simulink model "Tricopter_Controlled"  (R2012b)
settings: Solver=ode3  StartTime=0.0  StopTime=inf  FixedStep=T_sim  MaxStep=0.01  RelTol=1e-5
values from neighbouring files (symbols this model uses):
  A_l_max_x = sqrt( (Max_Thrust*3/m)^2  -  g^2  )    [Run3Copter.m]
  A_x = 0.015    [SetupComplete.m]
  A_y = A_x    (= 0.015)    [SetupComplete.m]
  A_z = 0.16    [SetupComplete.m]
  A_z_max = Max_Thrust*3/m    [Run3Copter.m]
  Alt_0 = input(' Give the initial altitude (m): ')    [Run3Copter.m]
  C_x = 1.2    [SetupComplete.m]
  C_y = C_x    (= 1.2)    [SetupComplete.m]
  C_z = 2.2    [SetupComplete.m]
  CG_0 = [0,0,0.02]'    [SetupComplete.m]
  epsilon = 0.01    [Run3Copter.m]
  eta_1 = deg2rad(-2)    [Run3Copter.m]
  eta_23 = 0    [Run3Copter.m]
  g = 9.81    [SetupComplete.m]
  h_M = 0.064    [SetupComplete.m]
  I_BAC_0 = [ Ix,0,Ixz;0,Iy,0;Ixz,0,Iz]    [SetupComplete.m]
  Initial_Omegas = Omega_hover    [Run3Copter.m]
  Initial_Torques = Torque_hover    [Run3Copter.m]
  Ix = 0.0552    [SetupComplete.m]
  Iy = 0.0552    [SetupComplete.m]
  Iz = 0.11    [SetupComplete.m]
  l = 0.345    [SetupComplete.m]
  l_arm = 0.264    [SetupComplete.m]
  latitude = 52.0733    [Run3Copter.m]
  longitude = 0.6278    [Run3Copter.m]
  m = 3.51    [SetupComplete.m]
  m_0 = 2.61    [SetupComplete.m]
  m_M = 0.300    (= 0.3)    [SetupComplete.m]
  rho = 1.15    [SetupComplete.m]
  Rotation_sign = [ 1,-1,-1]    [SetupComplete.m]
  T_sim = 0.01    [Run3Copter.m]
  throtle_1 = throtle_23/cos(eta_1)    [Run3Copter.m]
  throtle_23 = 0.745    [Run3Copter.m]
  v_i0 = sqrt( 1/3*m*g/(2*rho*pi*R^2)  )    [SetupComplete.m]
undefined symbols (not defined in the file or in its folder): DOWN_0, Earth, EAST_0, Newton, NORTH_0, P_0, Q_0, R_0, Raphson, U_0, V_0, W_0, WGS84
libraries: Adaptive_FaultTolerantControl x24, simulink_extras x11, XXCopter_C x7, XXCopter x5, aerolibfltsims x3, XXCopter_Control x2, qcatlib x1, aerolibconvert2 x1, aerolibtransform2 x1, aerolibanimutils x1, aerolibobsolete x1, simulink x1
(part 2 of 3)

== system Tricopter_Controlled/Inner Controller/P Controller ==
  note: These limits are wrong?
  note: Limits here for the maximum asymetrical thortle deflection
  Accels ref (m/s^2) : Inport
  Phi_ref (rad) : Inport  Port=2
  Theta_ref (rad) : Inport  Port=3
  Yaw_ref (rad) : Inport  Port=4
  All meas : Inport  Port=5
  Attitude Controller : Subsystem
  Body Rates Controller : Subsystem
  Bus Selector : BusSelector  OutputSignals=Meas.Euler meas (rad)
  Demux : Demux  Outputs=3
  MATLAB Function : MATLAB Function  TreatAsAtomicUnit=on
      settings: PermitHierarchicalResolution=ParametersOnly
  Mux : Mux  Inputs=2
  Saturation : Saturate  UpperLimit=[0.4,0.4,0.1]'  LowerLimit=-[0.4,0.4,0.1]'
  Saturation1 : Saturate  UpperLimit=deg2rad(45)/5*[2,2,1]'  LowerLimit=-deg2rad(45)/5*[2,2,1]'
  Accs_Ang_acc des : Outport
  wires:
  Accels ref (m/s^2)/1 -> Mux/1
  Body Rates Controller/1(Angular acc des (rad/s^2)) -> Saturation/1
  MATLAB Function/1(Omega) -> Demux/1
  Mux/1 -> Accs_Ang_acc des/1
  Attitude Controller/1(Euler_dot des (rad/s)) -> Saturation1/1
  All meas/1 -> Attitude Controller/4(All_meas), Body Rates Controller/4(All_meas), Bus Selector/1
  Phi_ref (rad)/1 -> Attitude Controller/1(phi_ref)
  Yaw_ref (rad)/1 -> Attitude Controller/3(psi_ref)
  Theta_ref (rad)/1 -> Attitude Controller/2(theta_ref)
  Bus Selector/1 -> MATLAB Function/2(euler_ang)  "<Euler meas (rad)>"
  Demux/1 -> Body Rates Controller/1(p_ref)
  Demux/2 -> Body Rates Controller/2(q_ref)
  Demux/3 -> Body Rates Controller/3(r_ref)
  Saturation/1 -> Mux/2
  Saturation1/1 -> MATLAB Function/1(ang_dot)

== system Tricopter_Controlled/Inner Controller/PI Controller ==
  note: Limits here for the maximum asymetrical thortle deflection
  Accels ref (m/s^2) : Inport
  Phi_ref (rad) : Inport  Port=2
  Theta_ref (rad) : Inport  Port=3
  Yaw_ref (rad) : Inport  Port=4
  All meas : Inport  Port=5
  Attitude Controller : Subsystem
  Body Rates Controller : Subsystem
  Bus Selector : BusSelector  OutputSignals=Meas.Euler meas (rad)
  Demux : Demux  Outputs=3
  Limits in Ang accel : Subsystem  TreatAsAtomicUnit=on
  MATLAB Function : MATLAB Function  TreatAsAtomicUnit=on
      settings: PermitHierarchicalResolution=ParametersOnly
  Mux : Mux  Inputs=2
  Saturation1 : Saturate  UpperLimit=deg2rad(45)*[1,1,0.5]'  LowerLimit=-deg2rad(45)*[1,1,0.5]'
  keep -pi/pi1 : Subsystem
  keep -pi/pi2 : Subsystem
  keep -pi/pi3 : Subsystem
  Accs_Ang_acc des : Outport
  wires:
  Limits in Ang accel/1(ang Ace des) -> Mux/2
  Demux/3 -> Body Rates Controller/3(r_ref)
  Demux/2 -> Body Rates Controller/2(q_ref)
  Demux/1 -> Body Rates Controller/1(p_ref)
  Bus Selector/1 -> Limits in Ang accel/2(Euler meas), MATLAB Function/2(euler_ang)  "<Euler meas (rad)>"
  Theta_ref (rad)/1 -> keep -pi/pi2/1(in (rad))
  Yaw_ref (rad)/1 -> keep -pi/pi3/1(in (rad))
  Phi_ref (rad)/1 -> keep -pi/pi1/1(in (rad))
  All meas/1 -> Body Rates Controller/4(All_meas), Bus Selector/1, Attitude Controller/4(All_meas)
  Mux/1 -> Accs_Ang_acc des/1
  MATLAB Function/1(Omega) -> Demux/1
  Accels ref (m/s^2)/1 -> Mux/1
  Body Rates Controller/1(Angular acc des (rad/s^2)) -> Limits in Ang accel/1(Ang Ace des)
  keep -pi/pi1/1(out (rad)) -> Attitude Controller/1(phi_ref)
  keep -pi/pi2/1(out (rad)) -> Attitude Controller/2(theta_ref)
  keep -pi/pi3/1(out (rad)) -> Attitude Controller/3(psi_ref)
  Attitude Controller/1(Euler_dot des (rad/s)) -> Saturation1/1
  Saturation1/1 -> MATLAB Function/1(ang_dot)

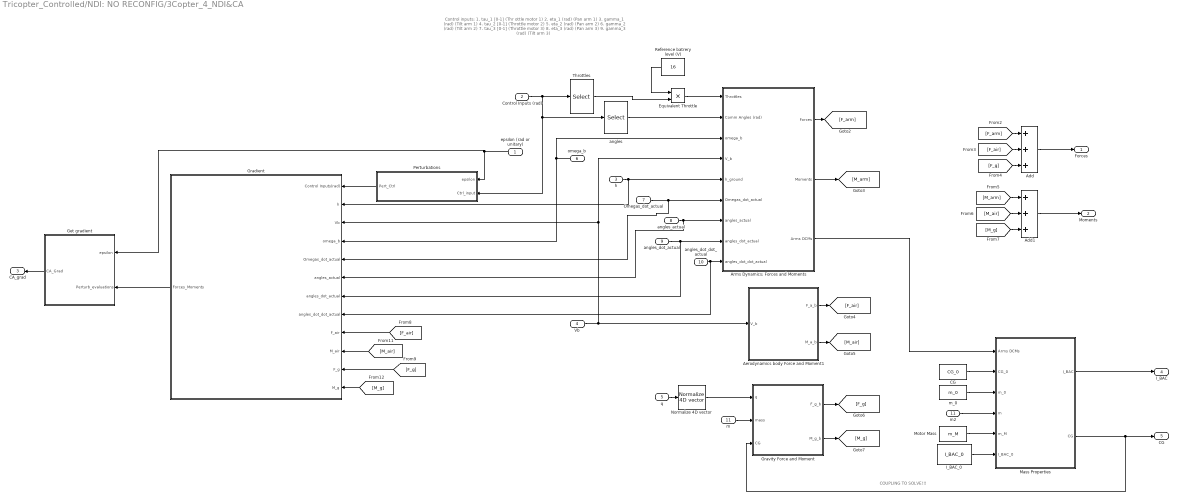
== system Tricopter_Controlled/NDI: NO RECONFIG/3Copter_4_NDI&CA ==
  note: Control inputs:
      | 1. tau_1 [0-1] (Thr ottle motor 1)
      | 2. eta_1 (rad)  (Pan arm 1)
      | 3. gamma_1 (rad)  (Tilt arm 1)
      |
      | 4. tau_2 [0-1] (Throttle motor 2)
      | 5. eta_2 (rad)  (Pan arm 2)
      | 6. gamma_2 (rad)  (Tilt arm 2)
      |
      | 7. tau_3 [0-1] (Throttle motor 3)
      | 8. eta_3 (rad)  (Pan arm  3)
      | 9. gamma_3 (rad)  (Tilt arm 3)
  note: COUPLING TO SOLVE!!!
  "epsilon (rad or unitary) " : Inport
  Control Inputs (rad) : Inport  Port=2
  h : Inport  Port=3
  Vb : Inport  Port=4
  q : Inport  Port=5
  omega_b : Inport  Port=6
  Omegas_dot_actual : Inport  Port=7
  angles_actual : Inport  Port=8
  angles_dot_actual : Inport  Port=9
  angles_dot_dot_actual : Inport  Port=10
  " m" : Inport  Port=11
  Add : Sum  Inputs=+++
  Add1 : Sum  Inputs=+++
  Aerodynamics body Force and Moment1 : MATLAB Function  TreatAsAtomicUnit=on
      settings: PermitHierarchicalResolution=ParametersOnly
  Arms Dynamics: Forces and Moments : Subsystem  TreatAsAtomicUnit=on
  CG : Constant  Value=CG_0
  Equivalent Throttle : Product  Inputs=**
  Get gradient : MATLAB Function  TreatAsAtomicUnit=on
      settings: PermitHierarchicalResolution=ParametersOnly
  Gradient : Subsystem  TreatAsAtomicUnit=on
  Gravity Force and Moment : MATLAB Function  TreatAsAtomicUnit=on
      settings: PermitHierarchicalResolution=ParametersOnly
  I_BAC_0 : Constant  Value=I_BAC_0
  Mass Properties : Subsystem  TreatAsAtomicUnit=on
  Motor Mass : Constant  Value=m_M
  Normalize 4D vector : XXCopter/Normalize 4D vector
  Perturbations : MATLAB Function  TreatAsAtomicUnit=on
      settings: PermitHierarchicalResolution=ParametersOnly
  Reference batrery level (V) : Constant  Value=16
  Throttles : Selector  IndexMode=Zero-based  InputPortWidth=9  Indices=[0,3,6]
  "angles " : Selector  IndexMode=Zero-based  InputPortWidth=9  Indices=[1,2,4,5,7,8]
  m2 : InportShadow  Port=11
  m_0 : Constant  Value=m_0
  Forces : Outport
  Moments : Outport  Port=2
  CA_grad : Outport  Port=3
  I_BAC : Outport  Port=4
  "CG " : Outport  Port=5
  wires:
  Get gradient/1(CA_Grad) -> CA_grad/1
  "epsilon (rad or unitary) "/1 -> Perturbations/1(epsilon), Get gradient/1(epsilon)
  Perturbations/1(Pert_Ctrl) -> Gradient/1("Control Inputs(rad) ")
  Gradient/1(Forces_Moments) -> Get gradient/2(Perturb_evaluations)
  Mass Properties/1(I_BAC) -> I_BAC/1
  [F_g] -> Gradient/11(F_g)
  [F_air] -> Gradient/9(F_air)
  [M_air] -> Gradient/10(M_air)
  [M_g] -> Gradient/12(M_g)
  Normalize 4D vector/1 -> Gravity Force and Moment/1(q)
  angles_dot_actual/1 -> Arms Dynamics: Forces and Moments/8(angles_dot_actual), Gradient/7(angles_dot_actual)
  Omegas_dot_actual/1 -> Gradient/5(Omegas_dot_actual), Arms Dynamics: Forces and Moments/6(Omegas_dot_actual)
  q/1 -> Normalize 4D vector/1
  Add1/1 -> Moments/1
  Reference batrery level (V)/1 -> Equivalent Throttle/1
  Equivalent Throttle/1 -> Arms Dynamics: Forces and Moments/1(Throttles)
  Mass Properties/2(CG) -> Gravity Force and Moment/3(CG), "CG "/1
  Add/1 -> Forces/1
  m2/1 -> Mass Properties/4(m)
  m_0/1 -> Mass Properties/3(m_0)
  I_BAC_0/1 -> Mass Properties/6(I_BAC_0)
  Motor Mass/1 -> Mass Properties/5(m_M)
  CG/1 -> Mass Properties/2(CG_0)
  Arms Dynamics: Forces and Moments/3(Arms DCMs) -> Mass Properties/1(Arms DCMs)
  Control Inputs (rad)/1 -> Throttles/1, Perturbations/2(Ctrl_input), "angles "/1
  Throttles/1 -> Equivalent Throttle/2
  [M_air] -> Add1/2
  [M_g] -> Add1/3
  [M_arm] -> Add1/1
  [F_g] -> Add/3
  [F_air] -> Add/2
  [F_arm] -> Add/1
  Gravity Force and Moment/2(M_g_b) -> [M_g]
  Gravity Force and Moment/1(F_g_b) -> [F_g]
  Aerodynamics body Force and Moment1/2(M_a_b) -> [M_air]
  Aerodynamics body Force and Moment1/1(F_a_b) -> [F_air]
  Arms Dynamics: Forces and Moments/2(Moments) -> [M_arm]
  Arms Dynamics: Forces and Moments/1(Forces) -> [F_arm]
  h/1 -> Gradient/2(h), Arms Dynamics: Forces and Moments/5(h_ground)
  " m"/1 -> Gravity Force and Moment/2(mass)
  omega_b/1 -> Gradient/4(omega_b), Arms Dynamics: Forces and Moments/3(omega_b)
  Vb/1 -> Aerodynamics body Force and Moment1/1(V_b), Arms Dynamics: Forces and Moments/4(V_b), Gradient/3(Vb)
  angles_actual/1 -> Gradient/6(angles_actual), Arms Dynamics: Forces and Moments/7(angles_actual)
  "angles "/1 -> Arms Dynamics: Forces and Moments/2(Comm Angles (rad))
  angles_dot_dot_actual/1 -> Gradient/8(angles_dot_dot_actual), Arms Dynamics: Forces and Moments/9(angles_dot_dot_actual)

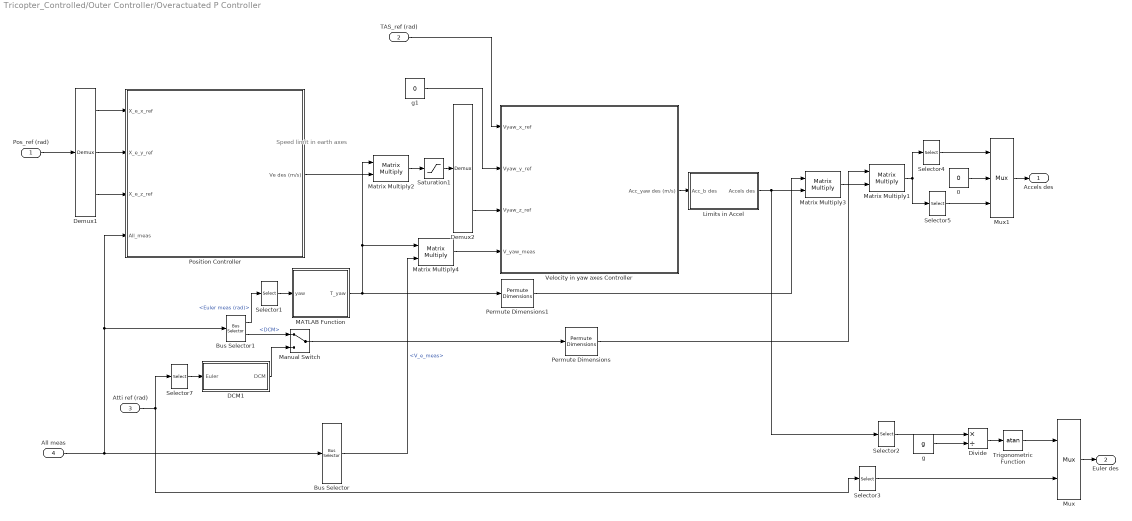
== system Tricopter_Controlled/Outer Controller/Overactuated P Controller ==
  note: Speed limit
      | in earth axes
  Pos_ref (rad) : Inport
  TAS_ref (rad) : Inport  Port=2
  Atti ref (rad) : Inport  Port=3
  All meas : Inport  Port=4
  0 : Constant  Value=0
  Bus Selector : BusSelector  OutputSignals=Meas.V_e_meas
  Bus Selector1 : BusSelector  OutputSignals=Meas.Euler meas (rad),DCM
  DCM1 : Subsystem  TreatAsAtomicUnit=on
  Demux1 : Demux  Outputs=3
  Demux2 : Demux  Outputs=3
  Divide : Product  Inputs=*/
  Limits in Accel : Subsystem  TreatAsAtomicUnit=on
  MATLAB Function : MATLAB Function  TreatAsAtomicUnit=on
      settings: PermitHierarchicalResolution=ParametersOnly
  Manual Switch : ManualSwitch
  Matrix Multiply{1..4} (4 alike) : Product  Multiplication=Matrix(*)
  Mux : Mux  Inputs=2
  Mux1 : Mux  Inputs=3
  Permute Dimensions : PermuteDimensions
  Permute Dimensions1 : PermuteDimensions
  Position Controller : Subsystem
  Saturation1 : Saturate  UpperLimit=[10,10,v_i0]  LowerLimit=-[10,10,v_i0*2]
  Selector1 : Selector  InputPortWidth=3  Indices=3
  Selector2 : Selector  InputPortWidth=3  Indices=2
  Selector3 : Selector  InputPortWidth=3  Indices=[2,3]
  Selector4 : Selector  InputPortWidth=3
  Selector5 : Selector  InputPortWidth=3  Indices=3
  Selector7 : Selector  InputPortWidth=3  Indices=[3 2 1]
  Trigonometric Function : Trigonometry  Operator=atan
  Velocity in yaw axes Controller : Subsystem
  g : Constant  Value=g
  g1 : Constant  Value=0
  Accels des : Outport
  Euler des : Outport  Port=2
  wires:
  Demux2/3 -> Velocity in yaw axes Controller/3(Vyaw_z_ref)
  Atti ref (rad)/1 -> Selector3/1, Selector7/1
  All meas/1 -> Position Controller/4(All_meas), Bus Selector1/1, Bus Selector/1
  Pos_ref (rad)/1 -> Demux1/1
  Demux1/3 -> Position Controller/3(X_e_z_ref)
  Demux1/2 -> Position Controller/2(X_e_y_ref)
  Demux1/1 -> Position Controller/1(X_e_x_ref)
  Selector7/1 -> DCM1/1(Euler)
  DCM1/1(DCM) -> Manual Switch/2
  Bus Selector1/2 -> Manual Switch/1  "<DCM>"
  Velocity in yaw axes Controller/1(Acc_yaw des (m/s)) -> Limits in Accel/1(Acc_b des)
  Matrix Multiply1/1 -> Selector4/1, Selector5/1
  Manual Switch/1 -> Permute Dimensions/1
  Permute Dimensions/1 -> Matrix Multiply1/1
  Selector1/1 -> MATLAB Function/1(yaw)
  Bus Selector1/1 -> Selector1/1  "<Euler meas (rad)>"
  Position Controller/1(Ve des (m/s)) -> Matrix Multiply2/2
  Saturation1/1 -> Demux2/1
  Limits in Accel/1(Accels des) -> Selector2/1, Matrix Multiply3/2
  MATLAB Function/1(T_yaw) -> Permute Dimensions1/1, Matrix Multiply2/1, Matrix Multiply4/1
  Matrix Multiply2/1 -> Saturation1/1
  Matrix Multiply3/1 -> Matrix Multiply1/2
  Permute Dimensions1/1 -> Matrix Multiply3/1
  Matrix Multiply4/1 -> Velocity in yaw axes Controller/4(V_yaw_meas)
  Bus Selector/1 -> Matrix Multiply4/2  "<V_e_meas>"
  TAS_ref (rad)/1 -> Velocity in yaw axes Controller/1(Vyaw_x_ref)
  Selector2/1 -> Divide/1
  g/1 -> Divide/2
  Divide/1 -> Trigonometric Function/1
  Mux/1 -> Euler des/1
  Selector3/1 -> Mux/2
  Mux1/1 -> Accels des/1
  Selector4/1 -> Mux1/1
  Selector5/1 -> Mux1/3
  0/1 -> Mux1/2
  Trigonometric Function/1 -> Mux/1
  g1/1 -> Velocity in yaw axes Controller/2(Vyaw_y_ref)

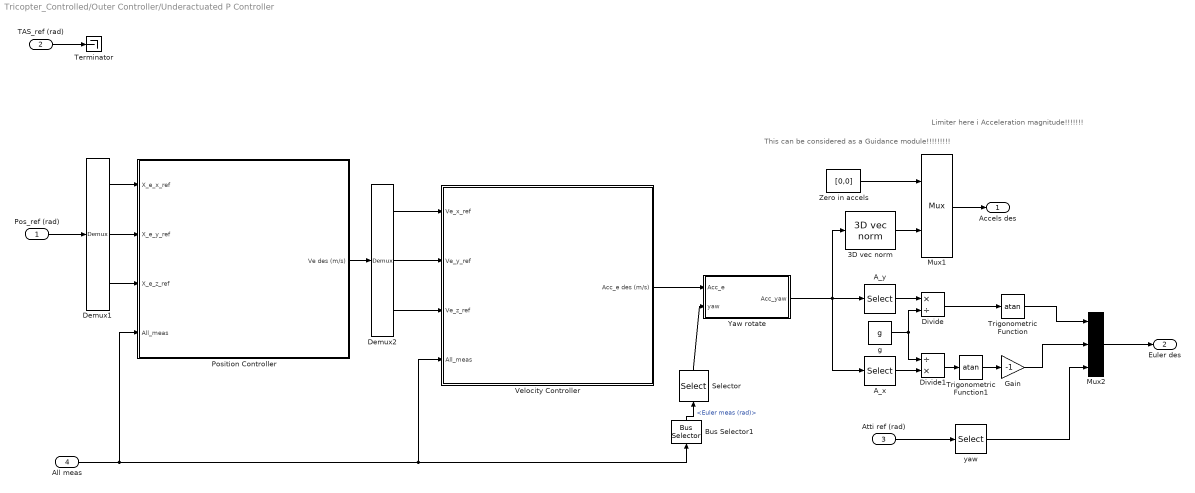
== system Tricopter_Controlled/Outer Controller/Underactuated P Controller ==
  note: This can be considered as a Guidance module!!!!!!!!!
  note: Limiter here i Acceleration magnitude!!!!!!!
  Pos_ref (rad) : Inport
  TAS_ref (rad) : Inport  Port=2
  Atti ref (rad) : Inport  Port=3
  All meas : Inport  Port=4
  3D vec norm : XXCopter_C/3D vec norm
  A_x : Selector  InputPortWidth=3
  A_y : Selector  InputPortWidth=3  Indices=2
  Bus Selector1 : BusSelector  OutputSignals=Meas.Euler meas (rad)
  Demux1 : Demux  Outputs=3
  Demux2 : Demux  Outputs=3
  Divide : Product  Inputs=*/
  Divide1 : Product  Inputs=/*
  Gain : Gain  Gain=-1
  Mux1 : Mux  Inputs=2
  Mux2 : Mux  Inputs=3
  Position Controller : Subsystem
  Selector : Selector  InputPortWidth=3  Indices=3
  Terminator : Terminator
  Trigonometric Function : Trigonometry  Operator=atan
  Trigonometric Function1 : Trigonometry  Operator=atan
  Velocity Controller : Subsystem
  Yaw rotate : MATLAB Function  TreatAsAtomicUnit=on
      settings: PermitHierarchicalResolution=ParametersOnly
  Zero in accels : Constant  Value=[0,0]
  g : Constant  Value=g
  yaw : Selector  InputPortWidth=3  Indices=3
  Accels des : Outport
  Euler des : Outport  Port=2
  wires:
  Zero in accels/1 -> Mux1/1
  Demux1/1 -> Position Controller/1(X_e_x_ref)
  Demux1/2 -> Position Controller/2(X_e_y_ref)
  Demux1/3 -> Position Controller/3(X_e_z_ref)
  Pos_ref (rad)/1 -> Demux1/1
  TAS_ref (rad)/1 -> Terminator/1
  All meas/1 -> Position Controller/4(All_meas), Velocity Controller/4(All_meas), Bus Selector1/1
  Mux2/1 -> Euler des/1
  Mux1/1 -> Accels des/1
  Position Controller/1(Ve des (m/s)) -> Demux2/1
  Demux2/2 -> Velocity Controller/2(Ve_y_ref)
  Demux2/1 -> Velocity Controller/1(Ve_x_ref)
  Demux2/3 -> Velocity Controller/3(Ve_z_ref)
  Velocity Controller/1(Acc_e des (m/s)) -> Yaw rotate/1(Acc_e)
  Bus Selector1/1 -> Selector/1  "<Euler meas (rad)>"
  Selector/1 -> Yaw rotate/2(yaw)
  3D vec norm/1 -> Mux1/2
  Yaw rotate/1(Acc_yaw) -> A_x/1, 3D vec norm/1, A_y/1
  Atti ref (rad)/1 -> yaw/1
  A_y/1 -> Divide/1
  g/1 -> Divide/2, Divide1/1
  A_x/1 -> Divide1/2
  Divide/1 -> Trigonometric Function/1
  Divide1/1 -> Trigonometric Function1/1
  Trigonometric Function1/1 -> Gain/1
  Trigonometric Function/1 -> Mux2/1
  Gain/1 -> Mux2/2
  yaw/1 -> Mux2/3

== system Tricopter_Controlled/Parameters estimation/DCM1 ==
  Euler : Inport  PortDimensions=3
  Fcn11 : Fcn  Expr=u(5)*u(4)
  Fcn12 : Fcn  Expr=u(5)*u(1)
  Fcn13 : Fcn  Expr=-u(2)
  Fcn21 : Fcn  Expr=u(3)*u(2)*u(4) - u(6)*u(1)
  Fcn22 : Fcn  Expr=u(3)*u(2)*u(1) + u(6)*u(4)
  Fcn23 : Fcn  Expr=u(3)*u(5)
  Fcn31 : Fcn  Expr=u(6)*u(2)*u(4) + u(3)*u(1)
  Fcn32 : Fcn  Expr=u(6)*u(2)*u(1) - u(3)*u(4)
  Fcn33 : Fcn  Expr=u(6)*u(5)
  Mux : Mux  Inputs=2
  Mux1 : Mux  Inputs=9
  Reshape : Reshape  OutputDimensionality=Customize  OutputDimensions=[3,3]
  sincos : Trigonometry  Operator=sincos
  DCM : Outport  PortDimensions=[3,3]
  wires:
  Fcn33/1 -> Mux1/9
  Fcn32/1 -> Mux1/8
  Fcn23/1 -> Mux1/6
  Fcn22/1 -> Mux1/5
  Fcn31/1 -> Mux1/7
  Fcn21/1 -> Mux1/4
  Fcn13/1 -> Mux1/3
  Fcn12/1 -> Mux1/2
  Fcn11/1 -> Mux1/1
  Mux/1 -> Fcn22/1, Fcn23/1, Fcn31/1, Fcn33/1, Fcn32/1, Fcn21/1, Fcn13/1, Fcn12/1, Fcn11/1
  sincos/2 -> Mux/2
  sincos/1 -> Mux/1
  Reshape/1 -> DCM/1
  Euler/1 -> sincos/1
  Mux1/1 -> Reshape/1

== system Tricopter_Controlled/3 Copter Complete/6dof Eqs of motion/DCM1 ==
  Euler : Inport  PortDimensions=3
  Fcn11 : Fcn  Expr=u(5)*u(4)
  Fcn12 : Fcn  Expr=u(5)*u(1)
  Fcn13 : Fcn  Expr=-u(2)
  Fcn21 : Fcn  Expr=u(3)*u(2)*u(4) - u(6)*u(1)
  Fcn22 : Fcn  Expr=u(3)*u(2)*u(1) + u(6)*u(4)
  Fcn23 : Fcn  Expr=u(3)*u(5)
  Fcn31 : Fcn  Expr=u(6)*u(2)*u(4) + u(3)*u(1)
  Fcn32 : Fcn  Expr=u(6)*u(2)*u(1) - u(3)*u(4)
  Fcn33 : Fcn  Expr=u(6)*u(5)
  Mux : Mux  Inputs=2
  Mux1 : Mux  Inputs=9
  Reshape : Reshape  OutputDimensionality=Customize  OutputDimensions=[3,3]
  sincos : Trigonometry  Operator=sincos
  DCM : Outport  PortDimensions=[3,3]
  wires:
  Fcn33/1 -> Mux1/9
  Fcn32/1 -> Mux1/8
  Fcn23/1 -> Mux1/6
  Fcn22/1 -> Mux1/5
  Fcn31/1 -> Mux1/7
  Fcn21/1 -> Mux1/4
  Fcn13/1 -> Mux1/3
  Fcn12/1 -> Mux1/2
  Fcn11/1 -> Mux1/1
  Mux/1 -> Fcn22/1, Fcn23/1, Fcn31/1, Fcn33/1, Fcn32/1, Fcn21/1, Fcn13/1, Fcn12/1, Fcn11/1
  sincos/2 -> Mux/2
  sincos/1 -> Mux/1
  Reshape/1 -> DCM/1
  Euler/1 -> sincos/1
  Mux1/1 -> Reshape/1

== system Tricopter_Controlled/3 Copter Complete/6dof Eqs of motion/q_dot ==
  note: Both of these methods to compute q_dot are very similar
  omega_b : Inport
  q : Inport  Port=2
  Quaternion_dot : MATLAB Function  TreatAsAtomicUnit=on  VariantObject=Variant
      settings: PermitHierarchicalResolution=ParametersOnly
  q_dot : Outport
  wires:
  omega_b/1 -> Quaternion_dot/1(omega_b)  "omega_b"
  q/1 -> Quaternion_dot/2(q)  "q"
  Quaternion_dot/1(q_dot) -> q_dot/1

== system Tricopter_Controlled/FlightGear visualization/Flat Earth to LLA/ne to lat//long ==
  Xe : Inport
  Demux : Demux  Outputs=2
  "Latitude Between +/- 90 " : Subsystem  TreatAsAtomicUnit=on
  "LongLat_offset " : Subsystem  TreatAsAtomicUnit=on
  "Longitude Between +/-180 " : Subsystem  TreatAsAtomicUnit=on
  Sel1 : Selector  InputPortWidth=3  Indices=[1,2]
  Sum2 : Sum  Inputs=++|
  initial_latg : Constant  Value=latitude
  initial_pos : Constant  Value=[latitude,longitude]
  rad2deg : Gain  Gain=180/pi  SaturateOnIntegerOverflow=on  OutDataTypeStr=Inherit: Same as input  ParamDataTypeStr=Inherit: Same as input
  lat_deg : Outport
  long_deg : Outport  Port=2
  wires:
  Xe/1 -> Sel1/1
  Sum2/1 -> "Latitude Between +/- 90 "/1(mu l)
  "LongLat_offset "/1(DeltaLL_rad) -> rad2deg/1
  Sel1/1 -> "LongLat_offset "/1(XY)
  rad2deg/1 -> Sum2/2
  initial_pos/1 -> Sum2/1
  initial_latg/1 -> "LongLat_offset "/2(mu)
  "Latitude Between +/- 90 "/1("mu l ") -> "Longitude Between +/-180 "/1(mu l)
  "Longitude Between +/-180 "/1("mu l ") -> Demux/1
  Demux/1 -> lat_deg/1
  Demux/2 -> long_deg/1

== system Tricopter_Controlled/Inner Controller/P Controller/Attitude Controller ==
  phi_ref : Inport
  theta_ref : Inport  Port=2
  psi_ref : Inport  Port=3
  All_meas : Inport  Port=4
  Bus Creator : BusCreator
  Bus Creator1 : BusCreator
  Bus Creator2 : BusCreator
  Bus Selector : BusSelector  OutputSignals=Meas.Euler meas (rad)
  Mux : Mux  Inputs=3
  Ref Model and P Controller p : Adaptive_FaultTolerantControl/Ref Model and P Controller  tau=1.5  y_i=0  K_f=1  K_b=2
  Ref Model and P Controller q : Adaptive_FaultTolerantControl/Ref Model and P Controller  tau=1.5  y_i=0  K_f=1  K_b=2
  Ref Model and P Controller q1 : Adaptive_FaultTolerantControl/Ref Model and P Controller  tau=5  y_i=0  K_f=0.5  K_b=1
  Selector : Selector  InputPortWidth=3
  Selector1 : Selector  InputPortWidth=3  Indices=2
  Selector2 : Selector  InputPortWidth=3  Indices=3
  Sum : Sum  Inputs=+-|
  Sum1 : Sum  Inputs=+-|
  Sum2 : Sum  Inputs=+-|
  Terminator1 : Terminator
  Terminator2 : Terminator
  Terminator3 : Terminator
  Euler_dot des (rad/s) : Outport
  wires:
  Ref Model and P Controller q1/4 -> Sum2/2
  Sum2/1 -> Bus Creator2/3  "Vz_err"
  Ref Model and P Controller q1/3 -> Bus Creator2/2, Sum2/1  "Vz_sf"
  Ref Model and P Controller q1/2 -> Bus Creator2/1  "Vz_sf_dot"
  Ref Model and P Controller q/5 -> Bus Creator1/4  "K_b_Vy"
  Ref Model and P Controller q/4 -> Sum1/2
  Sum1/1 -> Bus Creator1/3  "Vy_err"
  Ref Model and P Controller q/3 -> Bus Creator1/2, Sum1/1  "Vy_sf"
  Ref Model and P Controller q/2 -> Bus Creator1/1  "Vy_sf_dot"
  Ref Model and P Controller p/5 -> Bus Creator/4  "K_b_Vx"
  Ref Model and P Controller p/4 -> Sum/2
  Selector2/1 -> Ref Model and P Controller q1/2
  Bus Creator2/1 -> Terminator3/1
  Bus Creator1/1 -> Terminator1/1
  Bus Creator/1 -> Terminator2/1
  Sum/1 -> Bus Creator/3  "Vx_err"
  Ref Model and P Controller p/3 -> Bus Creator/2, Sum/1  "Vx_sf"
  Ref Model and P Controller p/2 -> Bus Creator/1  "Vx_sf_dot"
  Ref Model and P Controller q1/1 -> Mux/3
  Ref Model and P Controller q/1 -> Mux/2
  psi_ref/1 -> Ref Model and P Controller q1/1
  Selector1/1 -> Ref Model and P Controller q/2
  theta_ref/1 -> Ref Model and P Controller q/1
  Mux/1 -> Euler_dot des (rad/s)/1
  Ref Model and P Controller p/1 -> Mux/1
  Selector/1 -> Ref Model and P Controller p/2
  phi_ref/1 -> Ref Model and P Controller p/1
  Bus Selector/1 -> Selector2/1, Selector1/1, Selector/1  "<Euler meas (rad)>"
  All_meas/1 -> Bus Selector/1
  Ref Model and P Controller q1/5 -> Bus Creator2/4  "K_b_psi"

== system Tricopter_Controlled/Inner Controller/P Controller/Body Rates Controller ==
  p_ref : Inport
  q_ref : Inport  Port=2
  r_ref : Inport  Port=3
  All_meas : Inport  Port=4
  Bus Creator : BusCreator
  Bus Creator1 : BusCreator
  Bus Creator2 : BusCreator
  Bus Selector : BusSelector  OutputSignals=Meas.omega_b meas (rad/s)
  Mux : Mux  Inputs=3
  Ref Model and P Controller p : Adaptive_FaultTolerantControl/Ref Model and P Controller  tau=0.7  y_i=0  K_f=1  K_b=5
  Ref Model and P Controller q : Adaptive_FaultTolerantControl/Ref Model and P Controller  tau=0.7  y_i=0  K_f=1  K_b=5
  Ref Model and P Controller r : Adaptive_FaultTolerantControl/Ref Model and P Controller  tau=1.5  y_i=0  K_f=1  K_b=3
  Saturation : Saturate  UpperLimit=0.1  LowerLimit=-0.1
  Selector : Selector  InputPortWidth=3
  Selector1 : Selector  InputPortWidth=3  Indices=2
  Selector2 : Selector  InputPortWidth=3  Indices=3
  Sum : Sum  Inputs=+-|
  Sum1 : Sum  Inputs=+-|
  Sum2 : Sum  Inputs=+-|
  Terminator1 : Terminator
  Terminator2 : Terminator
  Terminator3 : Terminator
  Angular acc des (rad/s^2) : Outport
  wires:
  Ref Model and P Controller r/5 -> Bus Creator2/4  "K_b_r"
  Ref Model and P Controller r/4 -> Sum2/2
  Sum2/1 -> Bus Creator2/3  "r_err"
  Ref Model and P Controller r/3 -> Bus Creator2/2, Sum2/1  "r_sf"
  Ref Model and P Controller r/2 -> Bus Creator2/1  "r_sf_dot"
  Ref Model and P Controller q/5 -> Bus Creator1/4  "K_b_q"
  Ref Model and P Controller q/4 -> Sum1/2
  Sum1/1 -> Bus Creator1/3  "q_err"
  Ref Model and P Controller q/3 -> Bus Creator1/2, Sum1/1  "q_sf"
  Ref Model and P Controller q/2 -> Bus Creator1/1  "q_sf_dot"
  Ref Model and P Controller p/5 -> Bus Creator/4  "K_b_p"
  Ref Model and P Controller p/4 -> Sum/2
  Selector2/1 -> Ref Model and P Controller r/2
  Bus Creator2/1 -> Terminator3/1
  Bus Creator1/1 -> Terminator1/1
  Bus Creator/1 -> Terminator2/1
  Sum/1 -> Bus Creator/3  "p_err"
  Ref Model and P Controller p/3 -> Bus Creator/2, Sum/1  "p_sf"
  Ref Model and P Controller p/2 -> Bus Creator/1  "p_sf_dot"
  Ref Model and P Controller r/1 -> Saturation/1
  r_ref/1 -> Ref Model and P Controller r/1
  Selector1/1 -> Ref Model and P Controller q/2
  q_ref/1 -> Ref Model and P Controller q/1
  Mux/1 -> Angular acc des (rad/s^2)/1
  Selector/1 -> Ref Model and P Controller p/2
  p_ref/1 -> Ref Model and P Controller p/1
  Bus Selector/1 -> Selector2/1, Selector1/1, Selector/1  "<omega_b meas (rad/s)>"
  All_meas/1 -> Bus Selector/1
  Saturation/1 -> Mux/3
  Ref Model and P Controller q/1 -> Mux/2
  Ref Model and P Controller p/1 -> Mux/1

== system Tricopter_Controlled/Inner Controller/PI Controller/Attitude Controller ==
  phi_ref : Inport
  theta_ref : Inport  Port=2
  psi_ref : Inport  Port=3
  All_meas : Inport  Port=4
  Bus Creator : BusCreator
  Bus Creator1 : BusCreator
  Bus Creator2 : BusCreator
  Bus Selector : BusSelector  OutputSignals=Meas.Euler meas (rad)
  Mux : Mux  Inputs=3
  Ref Model and PI Controller : Adaptive_FaultTolerantControl/Ref Model and PI Controller  delta=0  tau=5  y_i=0  K_f=0  K_a=1  Con_way=pro  omega_n=4  xi=0.5  Z1=-30  K_b=1.5  f_i=0.1  f_c=1
  Ref Model and PI Controller1 : Adaptive_FaultTolerantControl/Ref Model and PI Controller  delta=0  tau=2  y_i=0  K_f=0  K_a=1  Con_way=pro  omega_n=4  xi=0.5  Z1=-30  K_b=3  f_i=0.1  f_c=1
  Ref Model and PI Controller2 : Adaptive_FaultTolerantControl/Ref Model and PI Controller  delta=0  tau=2  y_i=0  K_f=0  K_a=1  Con_way=pro  omega_n=4  xi=0.5  Z1=-30  K_b=3  f_i=0.1  f_c=1
  Selector : Selector  InputPortWidth=3
  Selector1 : Selector  InputPortWidth=3  Indices=2
  Selector2 : Selector  InputPortWidth=3  Indices=3
  Sum : Sum  Inputs=+-|
  Sum1 : Sum  Inputs=+-|
  Sum2 : Sum  Inputs=+-|
  Terminator1 : Terminator
  Terminator2 : Terminator
  Terminator3 : Terminator
  Euler_dot des (rad/s) : Outport
  wires:
  All_meas/1 -> Bus Selector/1
  Bus Selector/1 -> Selector1/1, Selector/1, Selector2/1  "<Euler meas (rad)>"
  phi_ref/1 -> Ref Model and PI Controller2/1
  Selector/1 -> Ref Model and PI Controller2/2
  Ref Model and PI Controller2/1 -> Mux/1
  Mux/1 -> Euler_dot des (rad/s)/1
  theta_ref/1 -> Ref Model and PI Controller1/1
  Selector1/1 -> Ref Model and PI Controller1/2
  psi_ref/1 -> Ref Model and PI Controller/1
  Ref Model and PI Controller1/1 -> Mux/2
  Ref Model and PI Controller/1 -> Mux/3
  Ref Model and PI Controller2/2 -> Bus Creator/1  "Vx_sf_dot"
  Ref Model and PI Controller2/3 -> Bus Creator/2, Sum/1  "Vx_sf"
  Sum/1 -> Bus Creator/3  "Vx_err"
  Bus Creator/1 -> Terminator2/1
  Bus Creator1/1 -> Terminator1/1
  Bus Creator2/1 -> Terminator3/1
  Selector2/1 -> Ref Model and PI Controller/2
  Ref Model and PI Controller2/4 -> Sum/2
  Ref Model and PI Controller1/2 -> Bus Creator1/1  "Vy_sf_dot"
  Ref Model and PI Controller1/3 -> Bus Creator1/2, Sum1/1  "Vy_sf"
  Sum1/1 -> Bus Creator1/3  "Vy_err"
  Ref Model and PI Controller1/4 -> Sum1/2
  Ref Model and PI Controller/2 -> Bus Creator2/1  "Vz_sf_dot"
  Ref Model and PI Controller/3 -> Sum2/1, Bus Creator2/2  "Vz_sf"
  Sum2/1 -> Bus Creator2/3  "Vz_err"
  Ref Model and PI Controller/4 -> Sum2/2

== system Tricopter_Controlled/Inner Controller/PI Controller/Body Rates Controller ==
  p_ref : Inport
  q_ref : Inport  Port=2
  r_ref : Inport  Port=3
  All_meas : Inport  Port=4
  Bus Creator : BusCreator
  Bus Creator1 : BusCreator
  Bus Creator2 : BusCreator
  Bus Selector : BusSelector  OutputSignals=Meas.omega_b meas (rad/s)
  Mux : Mux  Inputs=3
  Ref Model and P Controller p : Adaptive_FaultTolerantControl/Ref Model and P Controller  tau=0.7  y_i=0  K_f=0.7  K_b=2
  Ref Model and P Controller q : Adaptive_FaultTolerantControl/Ref Model and P Controller  tau=0.7  y_i=0  K_f=0.7  K_b=2
  Ref Model and P Controller r : Adaptive_FaultTolerantControl/Ref Model and P Controller  tau=1  y_i=0  K_f=0.5  K_b=1.5
  Saturation : Saturate  UpperLimit=0.1  LowerLimit=-0.1
  Selector : Selector  InputPortWidth=3
  Selector1 : Selector  InputPortWidth=3  Indices=2
  Selector2 : Selector  InputPortWidth=3  Indices=3
  Sum : Sum  Inputs=+-|
  Sum1 : Sum  Inputs=+-|
  Sum2 : Sum  Inputs=+-|
  Terminator1 : Terminator
  Terminator2 : Terminator
  Terminator3 : Terminator
  Angular acc des (rad/s^2) : Outport
  wires:
  Ref Model and P Controller p/1 -> Mux/1
  Ref Model and P Controller q/1 -> Mux/2
  Saturation/1 -> Mux/3
  All_meas/1 -> Bus Selector/1
  Bus Selector/1 -> Selector/1, Selector1/1, Selector2/1  "<omega_b meas (rad/s)>"
  p_ref/1 -> Ref Model and P Controller p/1
  Selector/1 -> Ref Model and P Controller p/2
  Mux/1 -> Angular acc des (rad/s^2)/1
  q_ref/1 -> Ref Model and P Controller q/1
  Selector1/1 -> Ref Model and P Controller q/2
  r_ref/1 -> Ref Model and P Controller r/1
  Ref Model and P Controller r/1 -> Saturation/1
  Ref Model and P Controller p/2 -> Bus Creator/1  "p_sf_dot"
  Ref Model and P Controller p/3 -> Sum/1, Bus Creator/2  "p_sf"
  Sum/1 -> Bus Creator/3  "p_err"
  Bus Creator/1 -> Terminator2/1
  Bus Creator1/1 -> Terminator1/1
  Bus Creator2/1 -> Terminator3/1
  Selector2/1 -> Ref Model and P Controller r/2
  Ref Model and P Controller p/4 -> Sum/2
  Ref Model and P Controller p/5 -> Bus Creator/4  "K_b_p"
  Ref Model and P Controller q/2 -> Bus Creator1/1  "q_sf_dot"
  Ref Model and P Controller q/3 -> Sum1/1, Bus Creator1/2  "q_sf"
  Sum1/1 -> Bus Creator1/3  "q_err"
  Ref Model and P Controller q/4 -> Sum1/2
  Ref Model and P Controller q/5 -> Bus Creator1/4  "K_b_q"
  Ref Model and P Controller r/2 -> Bus Creator2/1  "r_sf_dot"
  Ref Model and P Controller r/3 -> Sum2/1, Bus Creator2/2  "r_sf"
  Sum2/1 -> Bus Creator2/3  "r_err"
  Ref Model and P Controller r/4 -> Sum2/2
  Ref Model and P Controller r/5 -> Bus Creator2/4  "K_b_r"

== system Tricopter_Controlled/Inner Controller/PI Controller/Limits in Ang accel ==
  note: Here it is assumed that at all time every prop is generating m*g/3 newtons of force . It is conservative?
  Ang Ace des : Inport
  Euler meas : Inport  Port=2
  Limis eval : MATLAB Function  TreatAsAtomicUnit=on
      settings: PermitHierarchicalResolution=ParametersOnly
  Saturation Dynamic : simulink/Discontinuities/Saturation Dynamic  OutMin=[]  OutMax=[]  OutDataTypeStr=Inherit: Same as second input  OutDataType=fixdt(1, 16)  OutScaling=2^-10  DoSatur=off
  ang Ace des : Outport
  wires:
  Limis eval/1(Limit_up) -> Saturation Dynamic/1
  Limis eval/2(Limit_down) -> Saturation Dynamic/3
  Euler meas/1 -> Limis eval/2(euler_ang)
  Ang Ace des/1 -> Saturation Dynamic/2, Limis eval/1(Ang_Accel)
  Saturation Dynamic/1 -> ang Ace des/1

== system Tricopter_Controlled/Inner Controller/PI Controller/keep -pi//pi1 ==
  in (rad) : Inport
  Constant : Constant  Value=180
  Constant2 : Constant  Value=360
  Gain : Gain  Gain=360
  Math Function2 : Math  Operator=rem  SaturateOnIntegerOverflow=on
  Product : Product  Inputs=*/  RndMeth=Zero
  Rounding Function : Rounding  Operator=fix
  Sum2 : Sum  Inputs=|-+
  deg2rad1 : Gain  Gain=pi/180  SaturateOnIntegerOverflow=on  OutDataTypeStr=Inherit: Same as input  ParamDataTypeStr=Inherit: Same as input
  rad2deg : Gain  Gain=180/pi  SaturateOnIntegerOverflow=on  OutDataTypeStr=Inherit: Same as input  ParamDataTypeStr=Inherit: Same as input
  out (rad) : Outport
  wires:
  in (rad)/1 -> rad2deg/1
  Constant/1 -> Product/2
  Product/1 -> Rounding Function/1
  Rounding Function/1 -> Gain/1
  Gain/1 -> Sum2/1
  rad2deg/1 -> Math Function2/1
  Constant2/1 -> Math Function2/2
  Math Function2/1 -> Product/1, Sum2/2
  Sum2/1 -> deg2rad1/1
  deg2rad1/1 -> out (rad)/1

== system Tricopter_Controlled/Inner Controller/PI Controller/keep -pi//pi2 ==
  in (rad) : Inport
  Constant : Constant  Value=180
  Constant2 : Constant  Value=360
  Gain : Gain  Gain=360
  Math Function2 : Math  Operator=rem  SaturateOnIntegerOverflow=on
  Product : Product  Inputs=*/  RndMeth=Zero
  Rounding Function : Rounding  Operator=fix
  Sum2 : Sum  Inputs=|-+
  deg2rad1 : Gain  Gain=pi/180  SaturateOnIntegerOverflow=on  OutDataTypeStr=Inherit: Same as input  ParamDataTypeStr=Inherit: Same as input
  rad2deg : Gain  Gain=180/pi  SaturateOnIntegerOverflow=on  OutDataTypeStr=Inherit: Same as input  ParamDataTypeStr=Inherit: Same as input
  out (rad) : Outport
  wires:
  deg2rad1/1 -> out (rad)/1
  Sum2/1 -> deg2rad1/1
  Math Function2/1 -> Sum2/2, Product/1
  Constant2/1 -> Math Function2/2
  rad2deg/1 -> Math Function2/1
  Gain/1 -> Sum2/1
  Rounding Function/1 -> Gain/1
  Product/1 -> Rounding Function/1
  Constant/1 -> Product/2
  in (rad)/1 -> rad2deg/1

== system Tricopter_Controlled/Inner Controller/PI Controller/keep -pi//pi3 ==
  in (rad) : Inport
  Constant : Constant  Value=180
  Constant2 : Constant  Value=360
  Gain : Gain  Gain=360
  Math Function2 : Math  Operator=rem  SaturateOnIntegerOverflow=on
  Product : Product  Inputs=*/  RndMeth=Zero
  Rounding Function : Rounding  Operator=fix
  Sum2 : Sum  Inputs=|-+
  deg2rad1 : Gain  Gain=pi/180  SaturateOnIntegerOverflow=on  OutDataTypeStr=Inherit: Same as input  ParamDataTypeStr=Inherit: Same as input
  rad2deg : Gain  Gain=180/pi  SaturateOnIntegerOverflow=on  OutDataTypeStr=Inherit: Same as input  ParamDataTypeStr=Inherit: Same as input
  out (rad) : Outport
  wires:
  in (rad)/1 -> rad2deg/1
  Constant/1 -> Product/2
  Product/1 -> Rounding Function/1
  Rounding Function/1 -> Gain/1
  Gain/1 -> Sum2/1
  rad2deg/1 -> Math Function2/1
  Constant2/1 -> Math Function2/2
  Math Function2/1 -> Product/1, Sum2/2
  Sum2/1 -> deg2rad1/1
  deg2rad1/1 -> out (rad)/1

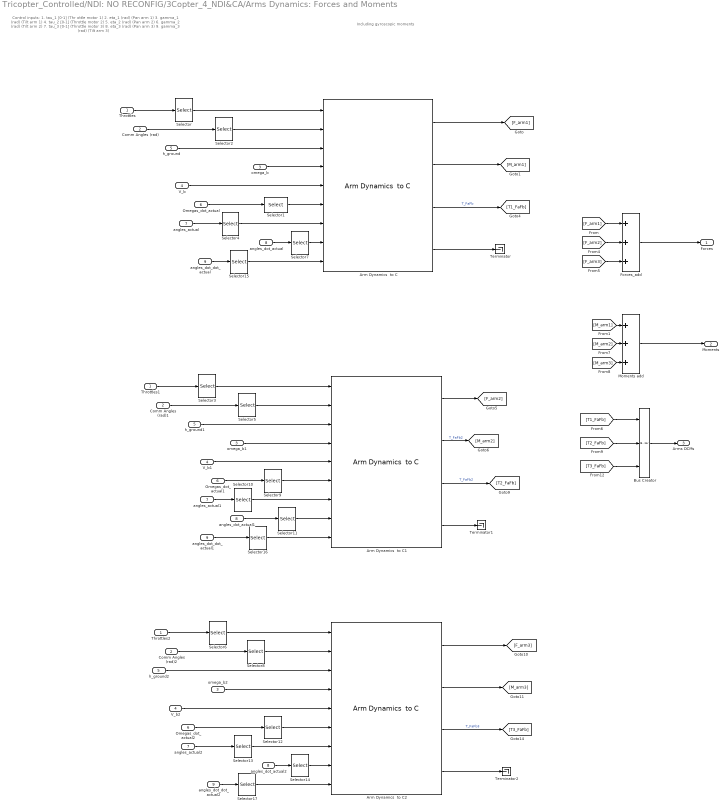
== system Tricopter_Controlled/NDI: NO RECONFIG/3Copter_4_NDI&CA/Arms Dynamics: Forces and Moments ==
  note: Including gyroscopic moments
  note: Control inputs:
      | 1. tau_1 [0-1] (Thr ottle motor 1)
      | 2. eta_1 (rad)  (Pan arm 1)
      | 3. gamma_1 (rad)  (Tilt arm 1)
      |
      | 4. tau_2 [0-1] (Throttle motor 2)
      | 5. eta_2 (rad)  (Pan arm 2)
      | 6. gamma_2 (rad)  (Tilt arm 2)
      |
      | 7. tau_3 [0-1] (Throttle motor 3)
      | 8. eta_3 (rad)  (Pan arm  3)
      | 9. gamma_3 (rad)  (Tilt arm 3)
  Throttles : Inport
  Comm Angles (rad) : Inport  Port=2
  omega_b : Inport  Port=3
  V_b : Inport  Port=4
  h_ground : Inport  Port=5
  Omegas_dot_actual : Inport  Port=6
  angles_actual : Inport  Port=7
  angles_dot_actual : Inport  Port=8
  angles_dot_dot_actual : Inport  Port=9
  Arm Dynamics  to C : XXCopter_C/Arm Dynamics  to C  Rot_sign=Rotation_sign(1)  arm_hub_pos=l*[1;0;0]  Arm_axis=[l_arm;0;0]  arm_num=1  eta_dir=[1;0;0]  gamma_dir=[0;1;0]  J_T=J_T  J_FA=J_FA  h=h  switch_val=direct_feedforward  omega_n=30  xi=1.4  eta_inf_lim=deg2rad(-180)  eta_sup_lim=deg2rad(180)  gamma_inf_lim=deg2rad(-90)  gamma_sup_lim=deg2rad(30)
  Arm Dynamics  to C1 : XXCopter_C/Arm Dynamics  to C  Rot_sign=Rotation_sign(2)  arm_hub_pos=l*[-1/2;sqrt(3)/2;0]  Arm_axis=[0;l_arm;0]  arm_num=2  eta_dir=[0;1;0]  gamma_dir=[1;0;0]  J_T=J_T  J_FA=J_FA  h=h  switch_val=direct_feedforward  omega_n=30  xi=1.4  eta_inf_lim=deg2rad(-180)  eta_sup_lim=deg2rad(180)  gamma_inf_lim=deg2rad(-30)  gamma_sup_lim=deg2rad(90)
  Arm Dynamics  to C2 : XXCopter_C/Arm Dynamics  to C  Rot_sign=Rotation_sign(3)  arm_hub_pos=l*[-1/2;-sqrt(3)/2;0]  Arm_axis=[0;-l_arm;0]  arm_num=3  eta_dir=[0;1;0]  gamma_dir=[1;0;0]  J_T=J_T  J_FA=J_FA  h=h  switch_val=direct_feedforward  omega_n=30  xi=1.4  eta_inf_lim=deg2rad(-180)  eta_sup_lim=deg2rad(180)  gamma_inf_lim=deg2rad(-90)  gamma_sup_lim=deg2rad(30)
  Bus Creator : BusCreator  Inputs=3
  Comm Angles (rad)1 : InportShadow  Port=2
  Comm Angles (rad)2 : InportShadow  Port=2
  Forces_add : Sum  Inputs=+++
  Moments add : Sum  Inputs=+++
  Omegas_dot_actual1 : InportShadow  Port=6
  Omegas_dot_actual2 : InportShadow  Port=6
  Selector : Selector  IndexMode=Zero-based  InputPortWidth=3  Indices=0
  Selector1 : Selector  IndexMode=Zero-based  InputPortWidth=3  Indices=0
  Selector{5,10..11,16} (4 alike) : Selector  IndexMode=Zero-based  InputPortWidth=6  Indices=[2,3]
  Selector12 : Selector  IndexMode=Zero-based  InputPortWidth=3  Indices=2
  Selector{8,13..14,17} (4 alike) : Selector  IndexMode=Zero-based  InputPortWidth=6  Indices=[4,5]
  Selector{2,4,7,15} (4 alike) : Selector  IndexMode=Zero-based  InputPortWidth=6  Indices=[0,1]
  Selector3 : Selector  IndexMode=Zero-based  InputPortWidth=3
  Selector6 : Selector  IndexMode=Zero-based  InputPortWidth=3  Indices=2
  Selector9 : Selector  IndexMode=Zero-based  InputPortWidth=3
  Terminator : Terminator
  Terminator1 : Terminator
  Terminator2 : Terminator
  Throttles1 : InportShadow
  Throttles2 : InportShadow
  V_b1 : InportShadow  Port=4
  V_b2 : InportShadow  Port=4
  angles_actual1 : InportShadow  Port=7
  angles_actual2 : InportShadow  Port=7
  angles_dot_actual1 : InportShadow  Port=8
  angles_dot_actual2 : InportShadow  Port=8
  angles_dot_dot_actual1 : InportShadow  Port=9
  angles_dot_dot_actual2 : InportShadow  Port=9
  h_ground1 : InportShadow  Port=5
  h_ground2 : InportShadow  Port=5
  omega_b1 : InportShadow  Port=3
  omega_b2 : InportShadow  Port=3
  Forces : Outport
  Moments : Outport  Port=2
  Arms DCMs : Outport  Port=3
  wires:
  Selector14/1 -> Arm Dynamics  to C2/8
  angles_actual2/1 -> Selector13/1
  angles_dot_actual2/1 -> Selector14/1
  Selector13/1 -> Arm Dynamics  to C2/7
  Selector12/1 -> Arm Dynamics  to C2/6
  Omegas_dot_actual2/1 -> Selector12/1
  Selector11/1 -> Arm Dynamics  to C1/8
  angles_actual1/1 -> Selector10/1
  angles_dot_actual1/1 -> Selector11/1
  Selector10/1 -> Arm Dynamics  to C1/7
  Selector9/1 -> Arm Dynamics  to C1/6
  Omegas_dot_actual1/1 -> Selector9/1
  Selector7/1 -> Arm Dynamics  to C/8
  angles_dot_actual/1 -> Selector7/1
  Selector4/1 -> Arm Dynamics  to C/7
  angles_actual/1 -> Selector4/1
  Selector1/1 -> Arm Dynamics  to C/6
  Omegas_dot_actual/1 -> Selector1/1
  [T3_FaFb] -> Bus Creator/3
  [T2_FaFb] -> Bus Creator/2
  [T1_FaFb] -> Bus Creator/1
  Bus Creator/1 -> Arms DCMs/1
  Arm Dynamics  to C1/2 -> [M_arm2]  "T_FaFb2"
  Arm Dynamics  to C1/1 -> [F_arm2]
  Arm Dynamics  to C2/4 -> Terminator2/1
  Arm Dynamics  to C1/4 -> Terminator1/1
  Arm Dynamics  to C/4 -> Terminator/1
  Arm Dynamics  to C2/3 -> [T3_FaFb]  "T_FaFb3"
  Comm Angles (rad)2/1 -> Selector8/1
  Selector8/1 -> Arm Dynamics  to C2/2
  omega_b2/1 -> Arm Dynamics  to C2/4
  Arm Dynamics  to C2/2 -> [M_arm3]
  Arm Dynamics  to C2/1 -> [F_arm3]
  h_ground2/1 -> Arm Dynamics  to C2/3
  V_b2/1 -> Arm Dynamics  to C2/5
  Selector6/1 -> Arm Dynamics  to C2/1
  Throttles2/1 -> Selector6/1
  Arm Dynamics  to C1/3 -> [T2_FaFb]  "T_FaFb2"
  Comm Angles (rad)1/1 -> Selector5/1
  Selector5/1 -> Arm Dynamics  to C1/2
  omega_b1/1 -> Arm Dynamics  to C1/4
  h_ground1/1 -> Arm Dynamics  to C1/3
  V_b1/1 -> Arm Dynamics  to C1/5
  Selector3/1 -> Arm Dynamics  to C1/1
  Throttles1/1 -> Selector3/1
  Arm Dynamics  to C/3 -> [T1_FaFb]  "T_FaFb"
  Comm Angles (rad)/1 -> Selector2/1
  Selector2/1 -> Arm Dynamics  to C/2
  [M_arm2] -> Moments add/2
  [M_arm3] -> Moments add/3
  [F_arm3] -> Forces_add/3
  [F_arm2] -> Forces_add/2
  omega_b/1 -> Arm Dynamics  to C/4
  [M_arm1] -> Moments add/1
  [F_arm1] -> Forces_add/1
  Arm Dynamics  to C/2 -> [M_arm1]
  Arm Dynamics  to C/1 -> [F_arm1]
  h_ground/1 -> Arm Dynamics  to C/3
  Moments add/1 -> Moments/1
  Forces_add/1 -> Forces/1
  V_b/1 -> Arm Dynamics  to C/5
  Selector/1 -> Arm Dynamics  to C/1
  Throttles/1 -> Selector/1
  angles_dot_dot_actual/1 -> Selector15/1
  Selector15/1 -> Arm Dynamics  to C/9
  angles_dot_dot_actual1/1 -> Selector16/1
  Selector16/1 -> Arm Dynamics  to C1/9
  angles_dot_dot_actual2/1 -> Selector17/1
  Selector17/1 -> Arm Dynamics  to C2/9

== system Tricopter_Controlled/NDI: NO RECONFIG/3Copter_4_NDI&CA/Gradient ==
  note: Control inputs:
      | 1. tau_1 [0-1] (Thr ottle motor 1)
      | 2. eta_1 (rad)  (Pan arm 1)
      | 3. gamma_1 (rad)  (Tilt arm 1)
      |
      | 4. tau_2 [0-1] (Throttle motor 2)
      | 5. eta_2 (rad)  (Pan arm 2)
      | 6. gamma_2 (rad)  (Tilt arm 2)
      |
      | 7. tau_3 [0-1] (Throttle motor 3)
      | 8. eta_3 (rad)  (Pan arm  3)
      | 9. gamma_3 (rad)  (Tilt arm 3)
  "Control Inputs(rad) " : Inport  Partition=on  PartitionDimension=1  PartitionWidth=9
  h : Inport  Port=2  Partition=off
  Vb : Inport  Port=3  Partition=off
  omega_b : Inport  Port=4  Partition=off
  Omegas_dot_actual : Inport  Port=5  Partition=off
  angles_actual : Inport  Port=6  Partition=off
  angles_dot_actual : Inport  Port=7  Partition=off
  angles_dot_dot_actual : Inport  Port=8  Partition=off
  F_air : Inport  Port=9  Partition=off
  M_air : Inport  Port=10  Partition=off
  F_g : Inport  Port=11  Partition=off
  M_g : Inport  Port=12  Partition=off
  Add : Sum  Inputs=+++
  Add1 : Sum  Inputs=+++
  Arms Dynamics: Forces and Moments : Subsystem  TreatAsAtomicUnit=on
  Equivalent Throttle : Product  Inputs=**
  For Each : ForEach  DisableCoverage=on  IndexMode=One-based
  Mux : Mux  Inputs=[3,3]
  Reference batrery level (V) : Constant  Value=16
  Signal Specification : SignalSpecification  Dimensions=[6,1]
  Terminator : Terminator
  Throttles : Selector  IndexMode=Zero-based  InputPortWidth=9  Indices=[0,3,6]
  "angles " : Selector  IndexMode=Zero-based  InputPortWidth=9  Indices=[1,2,4,5,7,8]
  Forces_Moments : Outport  ConcatenationDimension=2
  wires:
  Signal Specification/1 -> Forces_Moments/1
  Mux/1 -> Signal Specification/1
  Add1/1 -> Mux/2
  Add/1 -> Mux/1
  M_air/1 -> Add1/2
  M_g/1 -> Add1/3
  F_g/1 -> Add/3
  F_air/1 -> Add/2
  angles_dot_actual/1 -> Arms Dynamics: Forces and Moments/8(angles_dot_actual)
  Omegas_dot_actual/1 -> Arms Dynamics: Forces and Moments/6(Omegas_dot_actual)
  Reference batrery level (V)/1 -> Equivalent Throttle/1
  Equivalent Throttle/1 -> Arms Dynamics: Forces and Moments/1(Throttles)
  "Control Inputs(rad) "/1 -> "angles "/1, Throttles/1
  Throttles/1 -> Equivalent Throttle/2
  Arms Dynamics: Forces and Moments/1(Forces) -> Add/1
  h/1 -> Arms Dynamics: Forces and Moments/5(h_ground)
  omega_b/1 -> Arms Dynamics: Forces and Moments/3(omega_b)
  angles_actual/1 -> Arms Dynamics: Forces and Moments/7(angles_actual)
  "angles "/1 -> Arms Dynamics: Forces and Moments/2(Comm Angles (rad))
  angles_dot_dot_actual/1 -> Arms Dynamics: Forces and Moments/9(angles_dot_dot_actual)
  Arms Dynamics: Forces and Moments/2(Moments) -> Add1/1
  Arms Dynamics: Forces and Moments/3(Arms DCMs) -> Terminator/1
  Vb/1 -> Arms Dynamics: Forces and Moments/4(V_b)

== system Tricopter_Controlled/NDI: NO RECONFIG/3Copter_4_NDI&CA/Mass Properties ==
  Arms DCMs : Inport
  CG_0 : Inport  Port=2
  m_0 : Inport  Port=3
  m : Inport  Port=4
  m_M : Inport  Port=5
  I_BAC_0 : Inport  Port=6
  Arm Inertia : MATLAB Function  TreatAsAtomicUnit=on
      settings: PermitHierarchicalResolution=ParametersOnly
  Bus Selector : BusSelector  OutputSignals=T_FaFb,T_FaFb2,T_FaFb3
  CG position : Sum
  Divide : Product  Inputs=*/
  Divide1 : Product  Inputs=**
  Divide2 : Product  Inputs=/*
  Divide3 : Product  Inputs=**
  Motors Pos sum : Sum  Inputs=+++
  Total I_BAC : Sum
  I_BAC : Outport
  CG : Outport  Port=2
  wires:
  Arm Inertia/2(r1_M) -> Motors Pos sum/3
  I_BAC_0/1 -> Total I_BAC/1
  Arm Inertia/1(I_M) -> Total I_BAC/2
  Arm Inertia/4(r3_M) -> Motors Pos sum/1
  Arm Inertia/3(r2_M) -> Motors Pos sum/2
  Divide3/1 -> CG position/2
  Divide2/1 -> Divide3/2
  Motors Pos sum/1 -> Divide3/1
  Divide1/1 -> CG position/1
  CG position/1 -> CG/1
  m_M/1 -> Divide2/2
  Divide/1 -> Divide1/2
  CG_0/1 -> Divide1/1
  m/1 -> Divide2/1, Divide/2
  m_0/1 -> Divide/1
  Total I_BAC/1 -> I_BAC/1
  Bus Selector/1 -> Arm Inertia/1(T1_FAFb)  "<T_FaFb>"
  Bus Selector/2 -> Arm Inertia/2(T2_FAFb)  "<T_FaFb2>"
  Bus Selector/3 -> Arm Inertia/3(T3_FAFb)  "<T_FaFb3>"
  Arms DCMs/1 -> Bus Selector/1

== system Tricopter_Controlled/Outer Controller/Overactuated P Controller/DCM1 ==
  Euler : Inport  PortDimensions=3
  Fcn11 : Fcn  Expr=u(5)*u(4)
  Fcn12 : Fcn  Expr=u(5)*u(1)
  Fcn13 : Fcn  Expr=-u(2)
  Fcn21 : Fcn  Expr=u(3)*u(2)*u(4) - u(6)*u(1)
  Fcn22 : Fcn  Expr=u(3)*u(2)*u(1) + u(6)*u(4)
  Fcn23 : Fcn  Expr=u(3)*u(5)
  Fcn31 : Fcn  Expr=u(6)*u(2)*u(4) + u(3)*u(1)
  Fcn32 : Fcn  Expr=u(6)*u(2)*u(1) - u(3)*u(4)
  Fcn33 : Fcn  Expr=u(6)*u(5)
  Mux : Mux  Inputs=2
  Mux1 : Mux  Inputs=9
  Reshape : Reshape  OutputDimensionality=Customize  OutputDimensions=[3,3]
  sincos : Trigonometry  Operator=sincos
  DCM : Outport  PortDimensions=[3,3]
  wires:
  Fcn33/1 -> Mux1/9
  Fcn32/1 -> Mux1/8
  Fcn23/1 -> Mux1/6
  Fcn22/1 -> Mux1/5
  Fcn31/1 -> Mux1/7
  Fcn21/1 -> Mux1/4
  Fcn13/1 -> Mux1/3
  Fcn12/1 -> Mux1/2
  Fcn11/1 -> Mux1/1
  Mux/1 -> Fcn22/1, Fcn23/1, Fcn31/1, Fcn33/1, Fcn32/1, Fcn21/1, Fcn13/1, Fcn12/1, Fcn11/1
  sincos/2 -> Mux/2
  sincos/1 -> Mux/1
  Reshape/1 -> DCM/1
  Euler/1 -> sincos/1
  Mux1/1 -> Reshape/1

== system Tricopter_Controlled/Outer Controller/Overactuated P Controller/Limits in Accel ==
  note: Here limits apply by the maximum delfections and/or throtles.
      | Compute them!
  Acc_b des : Inport
  Saturation : Saturate  UpperLimit=[A_l_max_x,2,g]  LowerLimit=-[A_l_max_x,2,A_z_max-g]
  Accels des : Outport
  wires:
  Saturation/1 -> Accels des/1
  Acc_b des/1 -> Saturation/1

== system Tricopter_Controlled/Outer Controller/Overactuated P Controller/Position Controller ==
  X_e_x_ref : Inport
  X_e_y_ref : Inport  Port=2
  X_e_z_ref : Inport  Port=3
  All_meas : Inport  Port=4
  Bus Creator : BusCreator
  Bus Creator1 : BusCreator
  Bus Creator2 : BusCreator
  Bus Selector : BusSelector  OutputSignals=Meas.Pos meas (m)
  Mux : Mux  Inputs=3
  Ref Model and P Controller p : Adaptive_FaultTolerantControl/Ref Model and P Controller  tau=7  y_i=0  K_f=0  K_b=1
  Ref Model and P Controller q : Adaptive_FaultTolerantControl/Ref Model and P Controller  tau=7  y_i=0  K_f=0  K_b=1
  Ref Model and P Controller r : Adaptive_FaultTolerantControl/Ref Model and P Controller  tau=5  y_i=-Alt_0  K_f=0  K_b=2
  Selector : Selector  InputPortWidth=3
  Selector1 : Selector  InputPortWidth=3  Indices=2
  Selector2 : Selector  InputPortWidth=3  Indices=3
  Sum : Sum  Inputs=+-|
  Sum1 : Sum  Inputs=+-|
  Sum2 : Sum  Inputs=+-|
  Terminator1 : Terminator
  Terminator2 : Terminator
  Terminator3 : Terminator
  Ve des (m/s) : Outport
  wires:
  All_meas/1 -> Bus Selector/1
  Bus Selector/1 -> Selector/1, Selector1/1, Selector2/1  "<Pos meas (m)>"
  X_e_x_ref/1 -> Ref Model and P Controller p/1
  Selector/1 -> Ref Model and P Controller p/2
  Ref Model and P Controller p/1 -> Mux/1
  Mux/1 -> Ve des (m/s)/1
  X_e_y_ref/1 -> Ref Model and P Controller q/1
  Selector1/1 -> Ref Model and P Controller q/2
  X_e_z_ref/1 -> Ref Model and P Controller r/1
  Ref Model and P Controller q/1 -> Mux/2
  Ref Model and P Controller r/1 -> Mux/3
  Ref Model and P Controller p/2 -> Bus Creator/1  "X_ex_sf_dot"
  Ref Model and P Controller p/3 -> Sum/1, Bus Creator/2  "X_ex_sf"
  Sum/1 -> Bus Creator/3  "X_ex_err"
  Bus Creator/1 -> Terminator2/1
  Bus Creator1/1 -> Terminator1/1
  Bus Creator2/1 -> Terminator3/1
  Selector2/1 -> Ref Model and P Controller r/2
  Ref Model and P Controller p/4 -> Sum/2
  Ref Model and P Controller p/5 -> Bus Creator/4  "K_b_X_ex"
  Ref Model and P Controller q/2 -> Bus Creator1/1  "X_ey_sf_dot"
  Ref Model and P Controller q/3 -> Sum1/1, Bus Creator1/2  "X_e_y_sf"
  Sum1/1 -> Bus Creator1/3  "X_ey_err"
  Ref Model and P Controller q/4 -> Sum1/2
  Ref Model and P Controller q/5 -> Bus Creator1/4  "K_b_X_ey"
  Ref Model and P Controller r/2 -> Bus Creator2/1  "X_ez_sf_dot"
  Ref Model and P Controller r/3 -> Sum2/1, Bus Creator2/2  "X_ez_sf"
  Sum2/1 -> Bus Creator2/3  "X_ez_err"
  Ref Model and P Controller r/4 -> Sum2/2
  Ref Model and P Controller r/5 -> Bus Creator2/4  "K_b_X_e_z"

== system Tricopter_Controlled/Outer Controller/Overactuated P Controller/Velocity in yaw axes Controller ==
  Vyaw_x_ref : Inport
  Vyaw_y_ref : Inport  Port=2
  Vyaw_z_ref : Inport  Port=3
  V_yaw_meas : Inport  Port=4
  Bus Creator : BusCreator
  Bus Creator1 : BusCreator
  Bus Creator2 : BusCreator
  Mux : Mux  Inputs=3
  Ref Model and P Controller p : Adaptive_FaultTolerantControl/Ref Model and P Controller  tau=20  y_i=0  K_f=1  K_b=0.5
  Ref Model and P Controller q : Adaptive_FaultTolerantControl/Ref Model and P Controller  tau=5  y_i=0  K_f=0.5  K_b=0.8
  Ref Model and P Controller r : Adaptive_FaultTolerantControl/Ref Model and P Controller  tau=2  y_i=0  K_f=1  K_b=1
  Selector : Selector  InputPortWidth=3
  Selector1 : Selector  InputPortWidth=3  Indices=2
  Selector2 : Selector  InputPortWidth=3  Indices=3
  Sum : Sum  Inputs=+-|
  Sum1 : Sum  Inputs=+-|
  Sum2 : Sum  Inputs=+-|
  Terminator1 : Terminator
  Terminator2 : Terminator
  Terminator3 : Terminator
  Acc_yaw des (m/s) : Outport
  wires:
  Ref Model and P Controller r/5 -> Bus Creator2/4  "K_b_Ve_z"
  Ref Model and P Controller r/4 -> Sum2/2
  Sum2/1 -> Bus Creator2/3  "Vez_err"
  Ref Model and P Controller r/3 -> Bus Creator2/2, Sum2/1  "Vez_sf"
  Ref Model and P Controller r/2 -> Bus Creator2/1  "Vez_sf_dot"
  Ref Model and P Controller q/5 -> Bus Creator1/4  "K_b_Vey"
  Ref Model and P Controller q/4 -> Sum1/2
  Sum1/1 -> Bus Creator1/3  "Vey_err"
  Ref Model and P Controller q/3 -> Bus Creator1/2, Sum1/1  "Ve_y_sf"
  Ref Model and P Controller q/2 -> Bus Creator1/1  "Vey_sf_dot"
  Ref Model and P Controller p/5 -> Bus Creator/4  "K_b_Vex"
  Ref Model and P Controller p/4 -> Sum/2
  Selector2/1 -> Ref Model and P Controller r/2
  Bus Creator2/1 -> Terminator3/1
  Bus Creator1/1 -> Terminator1/1
  Bus Creator/1 -> Terminator2/1
  Sum/1 -> Bus Creator/3  "Vex_err"
  Ref Model and P Controller p/3 -> Bus Creator/2, Sum/1  "Vex_sf"
  Ref Model and P Controller p/2 -> Bus Creator/1  "Vex_sf_dot"
  Ref Model and P Controller r/1 -> Mux/3
  Ref Model and P Controller q/1 -> Mux/2
  Vyaw_z_ref/1 -> Ref Model and P Controller r/1
  Selector1/1 -> Ref Model and P Controller q/2
  Vyaw_y_ref/1 -> Ref Model and P Controller q/1
  Mux/1 -> Acc_yaw des (m/s)/1
  Ref Model and P Controller p/1 -> Mux/1
  Selector/1 -> Ref Model and P Controller p/2
  Vyaw_x_ref/1 -> Ref Model and P Controller p/1
  V_yaw_meas/1 -> Selector2/1, Selector1/1, Selector/1
